simulink model "furutapendulumsim"  (R2018a)
settings: Solver=VariableStepAuto  StartTime=0.0  StopTime=10  RelTol=1e-3
values from neighbouring files (symbols this model uses):
  A = [0,1,0,0 ... (first row only)    [furutapendulum.m]    (also in furutapendulum2.m = double(A); furutapendulum3.m = double(A); furutapendulum3_.m = double(A); furutapendulum4.m = double(A))
  B = [0 ... (first row only)    [furutapendulum.m]    (also in furutapendulum2.m = double(B); furutapendulum3.m = double(B); furutapendulum3_.m = double(B); furutapendulum4.m = double(B))
  length_base = 10e-3    (= 0.01)    [furutapendulum2.m]    (also in furutapendulum3.m; furutapendulum4.m)
  length_vert_cylinder = 200e-3    (= 0.2)    [furutapendulum2.m]    (also in furutapendulum3.m; furutapendulum4.m)
  m = 3.3e-3    (= 0.0033)    [furutapendulum2.m]    (also in furutapendulum3.m; furutapendulum4.m)
  radius_vert_cylinder = 10e-3    (= 0.01)    [furutapendulum2.m]    (also in furutapendulum3.m; furutapendulum4.m)
  s = tf('s')    [furutapendulum2.m]    (also in furutapendulum3.m; furutapendulum3_.m; furutapendulum4.m)
  Ts = 0.01    [furutapendulum2.m]    (also in furutapendulum3.m; furutapendulum4.m = 0.02)
undefined symbols (not defined in the file or in its folder): A1, A2, B1, B2, C1, C2, D1, D2, X, Y, Z
libraries: sm_lib x432, nesl_utility x54, cstblocks x15, aerolibanimutils x9, simulink x3
(part 13 of 13)

== system furutapendulumsim/Subsystem2/Plant2/h_RIP_pendulum_1_RIGID/h_connector_straight_1_RIGID ==
  Solid : sm_lib/Body Elements/Solid  InertiaType=Custom  Mass=0.00043271308549453917  MassUnits=kg  CenterOfMass=[8.0000017249971691 0 0]  CenterOfMassUnits=mm  MomentsOfInertia=[0.0031783748060293278 0.010562783552465226 0.010415546819518159]  MomentsOfInertiaUnits=kg*mm^2  ProductsOfInertia=[0 0 0]  ProductsOfInertiaUnits=kg*mm^2  DensityBased=on  Density=1000  DensityUnits=kg/(m^3)  DoExposeReferenceFrame=on  SerializedFrames=<Frames/>  GraphicType=FromGeometry  MarkerShape=Sphere  MarkerSize=10  MarkerSizeUnits=m  GraphicVisPropType=SimpleVisualProperties  GraphicDiffuseColor=[1 0 0]  GraphicSpecularColor=[0.5 0.5 0.5 1.0]  GraphicAmbientColor=[0.15 0.15 0.15 1.0]  GraphicEmissiveColor=[0.0 0.0 0.0 1.0]  GraphicShininess=75  GraphicOpacity=1  GeometryShape=FromFile  RectangleSize=[1 1]  RectangleSizeUnits=m  BrickDimensions=[1 1 1]  BrickDimensionUnits=m  CylinderRadius=1  CylinderRadiusUnits=m  CylinderLength=1  CylinderLengthUnits=m  SphereRadius=1  SphereRadiusUnits=m  EllipsoidRadii=[1 1 1]  EllipsoidRadiiUnits=m  ExtrusionCrossSection=[1 1; -1 1; -1 -1; 1 -1]  ExtrusionCrossSectionUnits=m  ExtrusionLength=1  ExtrusionLengthUnits=m  PolygonNumSides=3  PolygonOuterRadius=1  PolygonOuterRadiusUnits=m  ExtGeomFileType=STL  ExtGeomFileName=h_connector_straight_Default_sldprt.STL  ExtGeomFileUnits=mm  RevolutionCrossSection=[1 1; 1 -1; 2 -1; 2 1]  RevolutionCrossSectionUnits=m  RevolutionExtent=Full  RevolutionAngle=180  RevolutionAngleUnits=deg
  F : PMIOPort  Side=Left
  connections:
  Solid/RConn1 -- F/RConn1

== system furutapendulumsim/Subsystem2/Plant2/h_RIP_pendulum_1_RIGID/h_connector_straight_1_RIGID1 ==
  Solid : sm_lib/Body Elements/Solid  InertiaType=Custom  Mass=0.00043271308549453917  MassUnits=kg  CenterOfMass=[8.0000017249971691 0 0]  CenterOfMassUnits=mm  MomentsOfInertia=[0.0031783748060293278 0.010562783552465226 0.010415546819518159]  MomentsOfInertiaUnits=kg*mm^2  ProductsOfInertia=[0 0 0]  ProductsOfInertiaUnits=kg*mm^2  DensityBased=on  Density=1000  DensityUnits=kg/(m^3)  DoExposeReferenceFrame=on  SerializedFrames=<Frames/>  GraphicType=FromGeometry  MarkerShape=Sphere  MarkerSize=10  MarkerSizeUnits=m  GraphicVisPropType=SimpleVisualProperties  GraphicDiffuseColor=[1 0 0]  GraphicSpecularColor=[0.5 0.5 0.5 1.0]  GraphicAmbientColor=[0.15 0.15 0.15 1.0]  GraphicEmissiveColor=[0.0 0.0 0.0 1.0]  GraphicShininess=75  GraphicOpacity=1  GeometryShape=FromFile  RectangleSize=[1 1]  RectangleSizeUnits=m  BrickDimensions=[1 1 1]  BrickDimensionUnits=m  CylinderRadius=1  CylinderRadiusUnits=m  CylinderLength=1  CylinderLengthUnits=m  SphereRadius=1  SphereRadiusUnits=m  EllipsoidRadii=[1 1 1]  EllipsoidRadiiUnits=m  ExtrusionCrossSection=[1 1; -1 1; -1 -1; 1 -1]  ExtrusionCrossSectionUnits=m  ExtrusionLength=1  ExtrusionLengthUnits=m  PolygonNumSides=3  PolygonOuterRadius=1  PolygonOuterRadiusUnits=m  ExtGeomFileType=STL  ExtGeomFileName=h_connector_straight_Default_sldprt.STL  ExtGeomFileUnits=mm  RevolutionCrossSection=[1 1; 1 -1; 2 -1; 2 1]  RevolutionCrossSectionUnits=m  RevolutionExtent=Full  RevolutionAngle=180  RevolutionAngleUnits=deg
  F : PMIOPort  Side=Left
  connections:
  Solid/RConn1 -- F/RConn1

== system furutapendulumsim/Subsystem2/Plant2/h_encoderaxles_1_RIGID/connector_right_angle_1_RIGID ==
  Solid : sm_lib/Body Elements/Solid  InertiaType=Custom  Mass=0.00058767552757679601  MassUnits=kg  CenterOfMass=[-9.2850739875563288 3.0093098119265674e-05 2.6118746961723436]  CenterOfMassUnits=mm  MomentsOfInertia=[0.01287493955128299 0.021139675931830724 0.012862519708781989]  MomentsOfInertiaUnits=kg*mm^2  ProductsOfInertia=[1.0581915796389266e-07 0.0040573015479247326 -2.6079178646368151e-08]  ProductsOfInertiaUnits=kg*mm^2  DensityBased=on  Density=1000  DensityUnits=kg/(m^3)  DoExposeReferenceFrame=on  SerializedFrames=<Frames/>  GraphicType=FromGeometry  MarkerShape=Sphere  MarkerSize=10  MarkerSizeUnits=m  GraphicVisPropType=SimpleVisualProperties  GraphicDiffuseColor=[0.2 0.2 0.2]  GraphicSpecularColor=[0.5 0.5 0.5 1.0]  GraphicAmbientColor=[0.15 0.15 0.15 1.0]  GraphicEmissiveColor=[0.0 0.0 0.0 1.0]  GraphicShininess=75  GraphicOpacity=1  GeometryShape=FromFile  RectangleSize=[1 1]  RectangleSizeUnits=m  BrickDimensions=[1 1 1]  BrickDimensionUnits=m  CylinderRadius=1  CylinderRadiusUnits=m  CylinderLength=1  CylinderLengthUnits=m  SphereRadius=1  SphereRadiusUnits=m  EllipsoidRadii=[1 1 1]  EllipsoidRadiiUnits=m  ExtrusionCrossSection=[1 1; -1 1; -1 -1; 1 -1]  ExtrusionCrossSectionUnits=m  ExtrusionLength=1  ExtrusionLengthUnits=m  PolygonNumSides=3  PolygonOuterRadius=1  PolygonOuterRadiusUnits=m  ExtGeomFileType=STL  ExtGeomFileName=h_connector_right_angle_Default_sldprt.STL  ExtGeomFileUnits=mm  RevolutionCrossSection=[1 1; 1 -1; 2 -1; 2 1]  RevolutionCrossSectionUnits=m  RevolutionExtent=Full  RevolutionAngle=180  RevolutionAngleUnits=deg
  F : PMIOPort  Side=Left
  connections:
  Solid/RConn1 -- F/RConn1

== system furutapendulumsim/Subsystem2/Plant2/h_encoderaxles_1_RIGID/glidewheel_encoder_2_RIGID ==
  Solid : sm_lib/Body Elements/Solid  InertiaType=Custom  Mass=0.012717581311371812  MassUnits=kg  CenterOfMass=[20 23.311862389290109 3.5000000000000004]  CenterOfMassUnits=mm  MomentsOfInertia=[2.4036537381786549 1.6085577350900775 3.9083512258925288]  MomentsOfInertiaUnits=kg*mm^2  ProductsOfInertia=[0 0 0]  ProductsOfInertiaUnits=kg*mm^2  DensityBased=on  Density=1000  DensityUnits=kg/(m^3)  DoExposeReferenceFrame=on  SerializedFrames=<Frames/>  GraphicType=FromGeometry  MarkerShape=Sphere  MarkerSize=10  MarkerSizeUnits=m  GraphicVisPropType=SimpleVisualProperties  GraphicDiffuseColor=[0.4 0.4 0.4]  GraphicSpecularColor=[0.5 0.5 0.5 1.0]  GraphicAmbientColor=[0.15 0.15 0.15 1.0]  GraphicEmissiveColor=[0.0 0.0 0.0 1.0]  GraphicShininess=75  GraphicOpacity=1  GeometryShape=FromFile  RectangleSize=[1 1]  RectangleSizeUnits=m  BrickDimensions=[1 1 1]  BrickDimensionUnits=m  CylinderRadius=1  CylinderRadiusUnits=m  CylinderLength=1  CylinderLengthUnits=m  SphereRadius=1  SphereRadiusUnits=m  EllipsoidRadii=[1 1 1]  EllipsoidRadiiUnits=m  ExtrusionCrossSection=[1 1; -1 1; -1 -1; 1 -1]  ExtrusionCrossSectionUnits=m  ExtrusionLength=1  ExtrusionLengthUnits=m  PolygonNumSides=3  PolygonOuterRadius=1  PolygonOuterRadiusUnits=m  ExtGeomFileType=STL  ExtGeomFileName=glidewheel_encoder_Default_sldprt.STL  ExtGeomFileUnits=mm  RevolutionCrossSection=[1 1; 1 -1; 2 -1; 2 1]  RevolutionCrossSectionUnits=m  RevolutionExtent=Full  RevolutionAngle=180  RevolutionAngleUnits=deg
  F : PMIOPort  Side=Left
  connections:
  Solid/RConn1 -- F/RConn1

== system furutapendulumsim/Subsystem2/Plant2/h_encoderaxles_1_RIGID/h_triangle_1_RIGID ==
  Solid : sm_lib/Body Elements/Solid  InertiaType=Custom  Mass=0.0010321252629775849  MassUnits=kg  CenterOfMass=[0 0 -7.5566061536848483]  CenterOfMassUnits=mm  MomentsOfInertia=[0.036987929193085974 0.14119048806599191 0.1060088988565826]  MomentsOfInertiaUnits=kg*mm^2  ProductsOfInertia=[0 0 0]  ProductsOfInertiaUnits=kg*mm^2  DensityBased=on  Density=1000  DensityUnits=kg/(m^3)  DoExposeReferenceFrame=on  SerializedFrames=<Frames/>  GraphicType=FromGeometry  MarkerShape=Sphere  MarkerSize=10  MarkerSizeUnits=m  GraphicVisPropType=SimpleVisualProperties  GraphicDiffuseColor=[0.2 0.2 0.2]  GraphicSpecularColor=[0.5 0.5 0.5 1.0]  GraphicAmbientColor=[0.15 0.15 0.15 1.0]  GraphicEmissiveColor=[0.0 0.0 0.0 1.0]  GraphicShininess=75  GraphicOpacity=1  GeometryShape=FromFile  RectangleSize=[1 1]  RectangleSizeUnits=m  BrickDimensions=[1 1 1]  BrickDimensionUnits=m  CylinderRadius=1  CylinderRadiusUnits=m  CylinderLength=1  CylinderLengthUnits=m  SphereRadius=1  SphereRadiusUnits=m  EllipsoidRadii=[1 1 1]  EllipsoidRadiiUnits=m  ExtrusionCrossSection=[1 1; -1 1; -1 -1; 1 -1]  ExtrusionCrossSectionUnits=m  ExtrusionLength=1  ExtrusionLengthUnits=m  PolygonNumSides=3  PolygonOuterRadius=1  PolygonOuterRadiusUnits=m  ExtGeomFileType=STL  ExtGeomFileName=h_triangle_Default_sldprt.STL  ExtGeomFileUnits=mm  RevolutionCrossSection=[1 1; 1 -1; 2 -1; 2 1]  RevolutionCrossSectionUnits=m  RevolutionExtent=Full  RevolutionAngle=180  RevolutionAngleUnits=deg
  F : PMIOPort  Side=Left
  connections:
  Solid/RConn1 -- F/RConn1

== system furutapendulumsim/Subsystem2/Plant2/h_encoderaxles_1_RIGID/x86_axle_4_RIGID ==
  Solid : sm_lib/Body Elements/Solid  InertiaType=Custom  Mass=0.0011644908507951884  MassUnits=kg  CenterOfMass=[0 0 0]  CenterOfMassUnits=mm  MomentsOfInertia=[0.0027714374516001608 0.7160611630059921 0.7160611630059921]  MomentsOfInertiaUnits=kg*mm^2  ProductsOfInertia=[0 0 0]  ProductsOfInertiaUnits=kg*mm^2  DensityBased=on  Density=1000  DensityUnits=kg/(m^3)  DoExposeReferenceFrame=on  SerializedFrames=<Frames/>  GraphicType=FromGeometry  MarkerShape=Sphere  MarkerSize=10  MarkerSizeUnits=m  GraphicVisPropType=SimpleVisualProperties  GraphicDiffuseColor=[0.4 0.4 0.4]  GraphicSpecularColor=[0.5 0.5 0.5 1.0]  GraphicAmbientColor=[0.15 0.15 0.15 1.0]  GraphicEmissiveColor=[0.0 0.0 0.0 1.0]  GraphicShininess=75  GraphicOpacity=1  GeometryShape=FromFile  RectangleSize=[1 1]  RectangleSizeUnits=m  BrickDimensions=[1 1 1]  BrickDimensionUnits=m  CylinderRadius=1  CylinderRadiusUnits=m  CylinderLength=1  CylinderLengthUnits=m  SphereRadius=1  SphereRadiusUnits=m  EllipsoidRadii=[1 1 1]  EllipsoidRadiiUnits=m  ExtrusionCrossSection=[1 1; -1 1; -1 -1; 1 -1]  ExtrusionCrossSectionUnits=m  ExtrusionLength=1  ExtrusionLengthUnits=m  PolygonNumSides=3  PolygonOuterRadius=1  PolygonOuterRadiusUnits=m  ExtGeomFileType=STL  ExtGeomFileName=86_axle_Default_sldprt.STL  ExtGeomFileUnits=mm  RevolutionCrossSection=[1 1; 1 -1; 2 -1; 2 1]  RevolutionCrossSectionUnits=m  RevolutionExtent=Full  RevolutionAngle=180  RevolutionAngleUnits=deg
  F : PMIOPort  Side=Left
  connections:
  Solid/RConn1 -- F/RConn1

== system furutapendulumsim/Subsystem2/Plant2/h_encoderaxles_1_RIGID/x86_axle_5_RIGID ==
  Solid : sm_lib/Body Elements/Solid  InertiaType=Custom  Mass=0.0011644908507951884  MassUnits=kg  CenterOfMass=[0 0 0]  CenterOfMassUnits=mm  MomentsOfInertia=[0.0027714374516001608 0.7160611630059921 0.7160611630059921]  MomentsOfInertiaUnits=kg*mm^2  ProductsOfInertia=[0 0 0]  ProductsOfInertiaUnits=kg*mm^2  DensityBased=on  Density=1000  DensityUnits=kg/(m^3)  DoExposeReferenceFrame=on  SerializedFrames=<Frames/>  GraphicType=FromGeometry  MarkerShape=Sphere  MarkerSize=10  MarkerSizeUnits=m  GraphicVisPropType=SimpleVisualProperties  GraphicDiffuseColor=[0.4 0.4 0.4]  GraphicSpecularColor=[0.5 0.5 0.5 1.0]  GraphicAmbientColor=[0.15 0.15 0.15 1.0]  GraphicEmissiveColor=[0.0 0.0 0.0 1.0]  GraphicShininess=75  GraphicOpacity=1  GeometryShape=FromFile  RectangleSize=[1 1]  RectangleSizeUnits=m  BrickDimensions=[1 1 1]  BrickDimensionUnits=m  CylinderRadius=1  CylinderRadiusUnits=m  CylinderLength=1  CylinderLengthUnits=m  SphereRadius=1  SphereRadiusUnits=m  EllipsoidRadii=[1 1 1]  EllipsoidRadiiUnits=m  ExtrusionCrossSection=[1 1; -1 1; -1 -1; 1 -1]  ExtrusionCrossSectionUnits=m  ExtrusionLength=1  ExtrusionLengthUnits=m  PolygonNumSides=3  PolygonOuterRadius=1  PolygonOuterRadiusUnits=m  ExtGeomFileType=STL  ExtGeomFileName=86_axle_Default_sldprt.STL  ExtGeomFileUnits=mm  RevolutionCrossSection=[1 1; 1 -1; 2 -1; 2 1]  RevolutionCrossSectionUnits=m  RevolutionExtent=Full  RevolutionAngle=180  RevolutionAngleUnits=deg
  F : PMIOPort  Side=Left
  connections:
  Solid/RConn1 -- F/RConn1

== system furutapendulumsim/Subsystem2/Plant2/h_encoderaxles_1_RIGID/x86_axle_6_RIGID ==
  Solid : sm_lib/Body Elements/Solid  InertiaType=Custom  Mass=0.0011644908507951884  MassUnits=kg  CenterOfMass=[0 0 0]  CenterOfMassUnits=mm  MomentsOfInertia=[0.0027714374516001608 0.7160611630059921 0.7160611630059921]  MomentsOfInertiaUnits=kg*mm^2  ProductsOfInertia=[0 0 0]  ProductsOfInertiaUnits=kg*mm^2  DensityBased=on  Density=1000  DensityUnits=kg/(m^3)  DoExposeReferenceFrame=on  SerializedFrames=<Frames/>  GraphicType=FromGeometry  MarkerShape=Sphere  MarkerSize=10  MarkerSizeUnits=m  GraphicVisPropType=SimpleVisualProperties  GraphicDiffuseColor=[0.4 0.4 0.4]  GraphicSpecularColor=[0.5 0.5 0.5 1.0]  GraphicAmbientColor=[0.15 0.15 0.15 1.0]  GraphicEmissiveColor=[0.0 0.0 0.0 1.0]  GraphicShininess=75  GraphicOpacity=1  GeometryShape=FromFile  RectangleSize=[1 1]  RectangleSizeUnits=m  BrickDimensions=[1 1 1]  BrickDimensionUnits=m  CylinderRadius=1  CylinderRadiusUnits=m  CylinderLength=1  CylinderLengthUnits=m  SphereRadius=1  SphereRadiusUnits=m  EllipsoidRadii=[1 1 1]  EllipsoidRadiiUnits=m  ExtrusionCrossSection=[1 1; -1 1; -1 -1; 1 -1]  ExtrusionCrossSectionUnits=m  ExtrusionLength=1  ExtrusionLengthUnits=m  PolygonNumSides=3  PolygonOuterRadius=1  PolygonOuterRadiusUnits=m  ExtGeomFileType=STL  ExtGeomFileName=86_axle_Default_sldprt.STL  ExtGeomFileUnits=mm  RevolutionCrossSection=[1 1; 1 -1; 2 -1; 2 1]  RevolutionCrossSectionUnits=m  RevolutionExtent=Full  RevolutionAngle=180  RevolutionAngleUnits=deg
  F : PMIOPort  Side=Left
  connections:
  Solid/RConn1 -- F/RConn1

== matlab function furutapendulumsim/Subsystem1/MATLAB Function1 ==
  settings: updateMethod=DISCRETE
  data: y input; u output; A1 input; B1 input; C1 input; D1 input; A2 input; B2 input; C2 input; D2 input
function u = MCU(y, A1, B1, C1, D1, A2, B2, C2, D2)

r=0;
uo=0;
persistent x1; %static float x1[] = 0; (in C).
persistent x2; %static float x2[] = 0; (in C).
persistent yo; %static float r = {0,0}; (in C).
if isempty(x1) && isempty(x2) && isempty(yo)
    x1=zeros(2,1);
    x2=zeros(2,1);
    yo=[y(1) 0];
end

%state space representation of the loop shaping controller.
x1_=A1*x1+B1*(r-(y(1)-yo(1)));
%u1=C1.*x1+D1*(r-(y(1)-yo(1))) + uo;
u1=(C1(1)*x1(1)+C1(2)*x1(2))+D1*(r-(y(1)-yo(1)))+uo;

x2_=A2*x2+B2*(u1-(-y(2)-yo(2)));
%u2=C2.*x1+D2*(u1-(-y(2)-yo(2))) + uo;
u2=(C2(1)*x2(1)+C2(2)*x2(2))+D2*(u1-(-y(2)-yo(2)))+uo;

if (u2 > 100)
    u2 = 100;
elseif (u2 < -100)
    u2 = -100;
end    

x1=x1_;
x2=x2_;
u=u2;

== matlab function furutapendulumsim/Subsystem2/nonlinearsys1/MATLAB Function ==
  data: x input; u input; f output
function f = f(x,u)

%constants
g=9.81;
J1=1.7e-5; L1=8.8e-2; b1=1e-6*0;
J2=4.29e-5; m2=3.8261e-3; l2=8.67e-2; b2=1e-5*0;
J0=J1+m2*L1^2;

f1=x(2);
f2=([-J2*b1,m2*L1*l2*cos(x(3))*b2,-J2^2*sin(2*x(3)),-J2*m2*L1*l2*cos(x(3))*sin(2*x(3))/2,J2*m2*L1*l2*sin(x(3))]*[x(2);x(4);x(2)*x(4);x(2)^2;x(4)^2]+[J2,-m2*L1*l2*cos(x(3)),m2^2*l2^2*L1*sin(2*x(3))/2]*[u;0;g])/(J0*J2+(J2*sin(x(3)))^2-(m2*L1*l2*cos(x(3)))^2);
f3=x(4);
f4=([m2*L1*l2*cos(x(3))*b1,-b2*(J0+J2*sin(x(3))^2),m2*L1*l2*J2*cos(x(3))*sin(2*x(3)),-sin(2*x(3))*(J0*J2+(J2*sin(x(3)))^2)/2,-(m2*L1*l2)^2*sin(2*x(3))/2]*[x(2);x(4);x(2)*x(4);x(2)^2;x(4)^2]+[-m2*L1*l2*cos(x(3)),J0+J2*sin(x(3))^2,-m2*l2*sin(x(3))*(J0+J2*sin(x(3))^2)]*[u;0;g])/(J0*J2+(J2*sin(x(3)))^2-(m2*L1*l2*cos(x(3)))^2);

f=[f1;f2;f3;f4];

% function f = f(x,u)
% 
% %constants
% g=9.81;
% J1=1.7e-5; L1=8.8e-2; b1=1e-6*0;
% J2=4.29e-5; m2=3.8261e-3; l2=8.67e-2; b2=1e-5*0;
% J0=J1+m2*L1^2;
% 
% f1=x(2);
% f2=([-J2*b1,m2*L1*l2*cos(x(3))*b2,-J2*m2*l2^2*sin(2*x(3)),-m2^2*L1*l2^3*cos(x(3))*sin(2*x(3))/2,J2*m2*L1*l2*sin(x(3))]*[x(2);x(4);x(2)*x(4);x(2)^2;x(4)^2]+[J2,-m2*L1*l2*cos(x(3)),m2^2*l2^2*L1*sin(2*x(3))/2]*[u;0;g])/(J0*J2+J2*m2*l2^2*sin(x(3))^2-(m2*L1*l2*cos(x(3)))^2);
% f3=x(4);
% f4=([m2*L1*l2*cos(x(3))*b1,-b2*(J0+m2*l2^2*sin(x(3))^2),m2^2*L1*l2^3*cos(x(3))*sin(2*x(3)),-sin(2*x(3))*(J0*m2*l2^2+(m2*l2^2*sin(x(3)))^2)/2,-(m2*L1*l2)^2*sin(2*x(3))/2]*[x(2);x(4);x(2)*x(4);x(2)^2;x(4)^2]+[-m2*L1*l2*cos(x(3)),J0+m2*l2^2*sin(x(3))^2,-m2*l2*sin(x(3))*(J0+m2*l2^2*sin(x(3))^2)]*[u;0;g])/(J0*J2+J2*m2*l2^2*sin(x(3))^2-(m2*L1*l2*cos(x(3)))^2);
% 
% f=[f1;f2;f3;f4];

== matlab function furutapendulumsim/Subsystem2/nonlinearsys1/MATLAB Function1 ==
  data: x input; u input; y output
function y = h(x,u)

y = [x(1);x(3)];

== matlab function furutapendulumsim/Subsystem/Controller1/MATLAB Function1 ==
  settings: updateMethod=DISCRETE
  data: y input; u output; A1 input; B1 input; C1 input; D1 input; A2 input; B2 input; C2 input; D2 input
function u = MCU(y, A1, B1, C1, D1, A2, B2, C2, D2)

r=0;
uo=0;
persistent x1; %static float x1[] = 0; (in C).
persistent x2; %static float x2[] = 0; (in C).
persistent yo; %static float r = {0,0}; (in C).
if isempty(x1) && isempty(x2) && isempty(yo)
    x1=zeros(2,1);
    x2=zeros(2,1);
    yo=[y(1) 0];
end

%state space representation of the loop shaping controller.
x1_=A1*x1+B1*(r-(y(1)-yo(1)));
%u1=C1.*x1+D1*(r-(y(1)-yo(1))) + uo;
u1=(C1(1)*x1(1)+C1(2)*x1(2))+D1*(r-(y(1)-yo(1)))+uo;

x2_=A2*x2+B2*(u1-(-y(2)-yo(2)));
%u2=C2.*x1+D2*(u1-(-y(2)-yo(2))) + uo;
u2=(C2(1)*x2(1)+C2(2)*x2(2))+D2*(u1-(-y(2)-yo(2)))+uo;

if (u2 > 100)
    u2 = 100;
elseif (u2 < -100)
    u2 = -100;
end    

x1=x1_;
x2=x2_;
u=u2;

== matlab function furutapendulumsim/Subsystem1/nonlinearsys1/MATLAB Function ==
  data: x input; u input; f output
function f = f(x,u)

%constants
g=9.81;
J1=1.7e-5; L1=8.8e-2; b1=1e-6*0;
J2=4.29e-5; m2=3.8261e-3; l2=8.67e-2; b2=1e-5*0;
J0=J1+m2*L1^2;

f1=x(2);
f2=([-J2*b1,m2*L1*l2*cos(x(3))*b2,-J2^2*sin(2*x(3)),-J2*m2*L1*l2*cos(x(3))*sin(2*x(3))/2,J2*m2*L1*l2*sin(x(3))]*[x(2);x(4);x(2)*x(4);x(2)^2;x(4)^2]+[J2,-m2*L1*l2*cos(x(3)),m2^2*l2^2*L1*sin(2*x(3))/2]*[u;0;g])/(J0*J2+(J2*sin(x(3)))^2-(m2*L1*l2*cos(x(3)))^2);
f3=x(4);
f4=([m2*L1*l2*cos(x(3))*b1,-b2*(J0+J2*sin(x(3))^2),m2*L1*l2*J2*cos(x(3))*sin(2*x(3)),-sin(2*x(3))*(J0*J2+(J2*sin(x(3)))^2)/2,-(m2*L1*l2)^2*sin(2*x(3))/2]*[x(2);x(4);x(2)*x(4);x(2)^2;x(4)^2]+[-m2*L1*l2*cos(x(3)),J0+J2*sin(x(3))^2,-m2*l2*sin(x(3))*(J0+J2*sin(x(3))^2)]*[u;0;g])/(J0*J2+(J2*sin(x(3)))^2-(m2*L1*l2*cos(x(3)))^2);

f=[f1;f2;f3;f4];

% function f = f(x,u)
% 
% %constants
% g=9.81;
% J1=1.7e-5; L1=8.8e-2; b1=1e-6*0;
% J2=4.29e-5; m2=3.8261e-3; l2=8.67e-2; b2=1e-5*0;
% J0=J1+m2*L1^2;
% 
% f1=x(2);
% f2=([-J2*b1,m2*L1*l2*cos(x(3))*b2,-J2*m2*l2^2*sin(2*x(3)),-m2^2*L1*l2^3*cos(x(3))*sin(2*x(3))/2,J2*m2*L1*l2*sin(x(3))]*[x(2);x(4);x(2)*x(4);x(2)^2;x(4)^2]+[J2,-m2*L1*l2*cos(x(3)),m2^2*l2^2*L1*sin(2*x(3))/2]*[u;0;g])/(J0*J2+J2*m2*l2^2*sin(x(3))^2-(m2*L1*l2*cos(x(3)))^2);
% f3=x(4);
% f4=([m2*L1*l2*cos(x(3))*b1,-b2*(J0+m2*l2^2*sin(x(3))^2),m2^2*L1*l2^3*cos(x(3))*sin(2*x(3)),-sin(2*x(3))*(J0*m2*l2^2+(m2*l2^2*sin(x(3)))^2)/2,-(m2*L1*l2)^2*sin(2*x(3))/2]*[x(2);x(4);x(2)*x(4);x(2)^2;x(4)^2]+[-m2*L1*l2*cos(x(3)),J0+m2*l2^2*sin(x(3))^2,-m2*l2*sin(x(3))*(J0+m2*l2^2*sin(x(3))^2)]*[u;0;g])/(J0*J2+J2*m2*l2^2*sin(x(3))^2-(m2*L1*l2*cos(x(3)))^2);
% 
% f=[f1;f2;f3;f4];

== matlab function furutapendulumsim/Subsystem1/nonlinearsys1/MATLAB Function1 ==
  data: x input; u input; y output
function y = h(x,u)

y = [x(1);x(3)];

== matlab function furutapendulumsim/nonlinearsys2/MATLAB Function ==
  data: x input; u input; f output
function f = f(x,u)

%constants
g=9.81;
J1=1.7e-5; L1=8.8e-2; b1=1e-6*0;
J2=4.29e-5; m2=3.8261e-3; l2=8.67e-2; b2=1e-5*0;
J0=J1+m2*L1^2;

f1=x(2);
f2=([-J2*b1,m2*L1*l2*cos(x(3))*b2,-J2^2*sin(2*x(3)),-J2*m2*L1*l2*cos(x(3))*sin(2*x(3))/2,J2*m2*L1*l2*sin(x(3))]*[x(2);x(4);x(2)*x(4);x(2)^2;x(4)^2]+[J2,-m2*L1*l2*cos(x(3)),m2^2*l2^2*L1*sin(2*x(3))/2]*[u;0;g])/(J0*J2+(J2*sin(x(3)))^2-(m2*L1*l2*cos(x(3)))^2);
f3=x(4);
f4=([m2*L1*l2*cos(x(3))*b1,-b2*(J0+J2*sin(x(3))^2),m2*L1*l2*J2*cos(x(3))*sin(2*x(3)),-sin(2*x(3))*(J0*J2+(J2*sin(x(3)))^2)/2,-(m2*L1*l2)^2*sin(2*x(3))/2]*[x(2);x(4);x(2)*x(4);x(2)^2;x(4)^2]+[-m2*L1*l2*cos(x(3)),J0+J2*sin(x(3))^2,-m2*l2*sin(x(3))*(J0+J2*sin(x(3))^2)]*[u;0;g])/(J0*J2+(J2*sin(x(3)))^2-(m2*L1*l2*cos(x(3)))^2);

f=[f1;f2;f3;f4];

% function f = f(x,u)
% 
% %constants
% g=9.81;
% J1=1.7e-5; L1=8.8e-2; b1=1e-6*0;
% J2=4.29e-5; m2=3.8261e-3; l2=8.67e-2; b2=1e-5*0;
% J0=J1+m2*L1^2;
% 
% f1=x(2);
% f2=([-J2*b1,m2*L1*l2*cos(x(3))*b2,-J2*m2*l2^2*sin(2*x(3)),-m2^2*L1*l2^3*cos(x(3))*sin(2*x(3))/2,J2*m2*L1*l2*sin(x(3))]*[x(2);x(4);x(2)*x(4);x(2)^2;x(4)^2]+[J2,-m2*L1*l2*cos(x(3)),m2^2*l2^2*L1*sin(2*x(3))/2]*[u;0;g])/(J0*J2+J2*m2*l2^2*sin(x(3))^2-(m2*L1*l2*cos(x(3)))^2);
% f3=x(4);
% f4=([m2*L1*l2*cos(x(3))*b1,-b2*(J0+m2*l2^2*sin(x(3))^2),m2^2*L1*l2^3*cos(x(3))*sin(2*x(3)),-sin(2*x(3))*(J0*m2*l2^2+(m2*l2^2*sin(x(3)))^2)/2,-(m2*L1*l2)^2*sin(2*x(3))/2]*[x(2);x(4);x(2)*x(4);x(2)^2;x(4)^2]+[-m2*L1*l2*cos(x(3)),J0+m2*l2^2*sin(x(3))^2,-m2*l2*sin(x(3))*(J0+m2*l2^2*sin(x(3))^2)]*[u;0;g])/(J0*J2+J2*m2*l2^2*sin(x(3))^2-(m2*L1*l2*cos(x(3)))^2);
% 
% f=[f1;f2;f3;f4];

== matlab function furutapendulumsim/nonlinearsys2/MATLAB Function1 ==
  data: x input; u input; y output
function y = h(x,u)

y = [x(1);x(3)];
